simulink model "SledUnit_Levitation_Control"  (R2025a)
settings: Solver=ode23t  StartTime=0.0  StopTime=T_sim  FixedStep=0.0001  RelTol=1e-3
PreLoadFcn:
  | setup_sim_params
model workspace: external: MATLAB File .\Setup_Machine_Model\setup_structure_params.m (data not in the file)
values from neighbouring files (symbols this model uses):
  N = numel(time)    [evaluation_sled_levitation.m]
  noise_switch = 1    [setup_sim_params.m]
undefined symbols (not defined in the file or in its folder): CartJointInit, obs_init_state, obs_params, SledUnitMass, ssc_params, SUInitPosAtt2SlGCS, X, Y, Z
libraries: sm_lib x51, nesl_utility x4
(part 1 of 3)
settings Model: NumberOfSteps=3  Creator=Polarstern  LastModifiedBy=CelestialAurora
settings DataIOCC: SaveOutput=off
settings ExplorerConfigSet: SimMechanicsOpenEditorOnUpdate=off
settings ExplorerConfigSet: InternalSimMechanicsExplorerSettings=|
  | <ExplorerConfiguration>
  | 
  |   <canonicalview>planar_xy</canonicalview>
  | 
  |   <TilePanel>
  |     <TileInfo>
  |       <Tiles Columns="1" Count="1" Height="608" Rows="1" Width="1079">
  |         <Row Weight="1"/>
  |         <Column Weight="1"/>
  |         <Tile Height="1" Width="1" X="0" Y="0"/>
  |       </Tiles>
  |     </TileInfo>
  |     <SceneInfo>
  |       <SceneViewer>
  |         <IsThisViewStd>
  |           <IsStandardView>off</IsStandardView>
  |           <StandardViewName>Front</StandardViewName>
  |         </IsThisViewStd>
  |         <BGColor>
  |           <R>1</R>
  |           <G>1</G>
  |           <B>1</B>
  |           <A>1</A>
  |         </BGColor>
  |         <Camera>
  |           <DoPerspective>off</DoPerspective>
  |           <Position>
  |             <X>0.093469102418852493</X>
  |             <Y>0.022043424721416197</Y>
  |             <Z>11.197877009761701</Z>
  |           </Position>
  |           <Center>
  |             <X>0.093469102418852493</X>
  |             <Y>0.022043424721416197</Y>
  |             <Z>1.2744981024265289</Z>
  |           </Center>
  |           <Up>
  |             <X>0</X>
  |             <Y>1</Y>
  |             <Z>0</Z>
  |           </Up>
  |           <XLim>0.23710801149158423</XLim>
  |           <YLim>0.23710801149158423</YLim>
  |           <ViewLimDist>0.01</ViewLimDist>
  |         </Camera>
  |       </SceneViewer>
  |     </SceneInfo>
  |   </TilePanel>
  | 
  |   <MechEditorPanel>
  |     <GfxPanelCameraMap/>
  |     <Cameras/>
  |     <VideoCreator>
  |       <IncludeTiles>All</IncludeTiles>
  |       <IncludeTime>on</IncludeTime>
  |       <IncludeWorldFrame>off</IncludeWorldFrame>
  |       <PlaybackSpeedRatio>1</PlaybackSpeedRatio>
  |       <FrameRate>30</FrameRate>
  |       <FrameSize>auto</FrameSize>
  |       <VideoFormat>UncompressedAVI</VideoFormat>
  |     </VideoCreator>
  |   </MechEditorPanel>
  | 
  |   <PlaybackSettings>
  |     <PlaybackSpeedFactor>0.25</PlaybackSpeedFactor>
  |   </PlaybackSettings>
  | 
  | </ExplorerConfiguration>

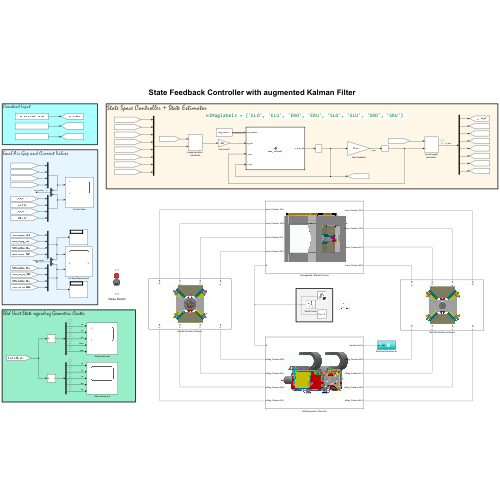
[thumbnail: Simulink's stored preview of the top-level diagram]
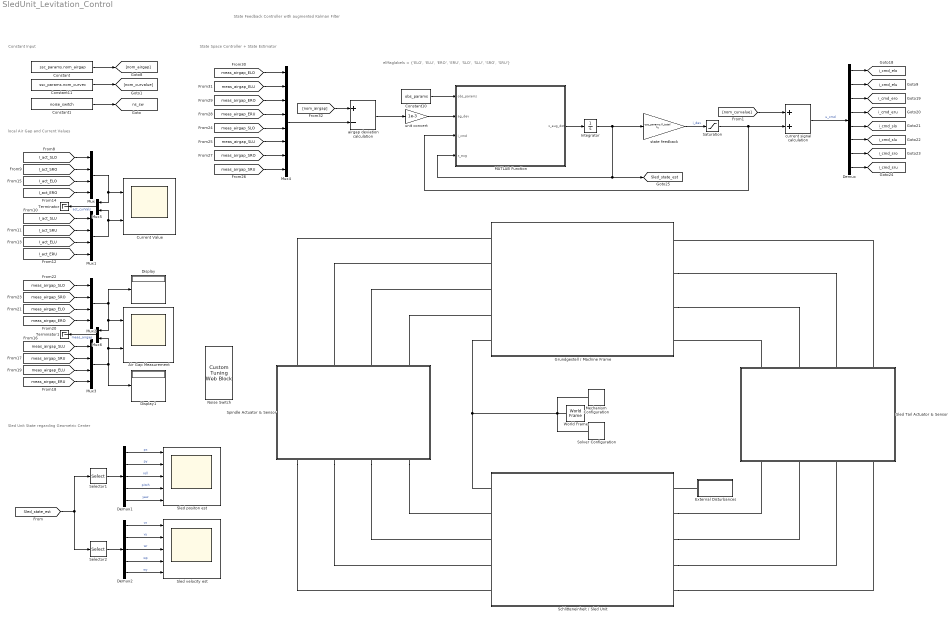
== system SledUnit_Levitation_Control ==
  note: Sled Unit State regarding Geometric Center
  note: State Space Controller + State Estimator
  note: elMaglabels = {'ELO', 'ELU', 'ERO', 'ERU', 'SLO', 'SLU', 'SRO', 'SRU'}
  note: Constant Input
  note: local Air Gap and Current Values
  note: State Feedback Controller with augmented Kalman Filter
  Air Gap Measurement : Scope  NumInputPorts=2
      settings: ActiveDisplayYMinimum=0.43274901204317934  ActiveDisplayYMaximum=0.52575342044124662  YLabel=mm
  Constant : Constant  Value=ssc_params.nom_airgap
  Constant1 : Constant  Value=noise_switch
  Constant10 : Constant  Value=obs_params  OutDataTypeStr=Bus: obs_Bus
  Constant11 : Constant  Value=ssc_params.nom_curvec
  Current Value : Scope  NumInputPorts=2
      settings: ActiveDisplayYMinimum=8.21336168307043  ActiveDisplayYMaximum=15.633373377132628
  Demux : Demux  Outputs=8
  Demux1 : Demux  Outputs=5
  Demux2 : Demux  Outputs=5
  Display : Display
  Display1 : Display
  External Disturbances : Subsystem
  Grundgestell / Machine Frame : Subsystem
      mask Display: image('.\BlockMaskIcons\machine_stand.png', [0,0,0,0,70,70]);
  Integrator : Integrator  InitialCondition=obs_init_state
  MATLAB Function : MATLAB Function  TreatAsAtomicUnit=on
  Mechanism Configuration : sm_lib/Utilities/Mechanism Configuration  UniformGravity=Constant  GravityVector=grav  GravityVectorUnits=m/s^2  LinearizationDelta=0.001  JointModeTransitionNonlinearIterations=2
  Mux{,1..3} (4 alike) : Mux
  Mux4 : Mux  Inputs=8
  Mux5 : Mux  Inputs=2
  Mux6 : Mux  Inputs=2
  Noise Switch : CustomTuningWebBlock  LabelPosition=Hide  ShowInitialText=on  Configuration="{\"components\":[{\"name\":\"CustomSwitchStateComponent\",\"settings\":{\"position\":[0,0,1,1],\"showAllLabels\":1,\"states\":[{\"HitRegion\":{\"position\":[0.5,0,1,0.5]},\"Image\":{\"position\":[0,0.24928571428571428,0.5014285714285714,1],\"size\":[0.5014285714285714,1],\"src\":\"data:image\\/svg+xml;base64,PHN2ZyB4bWxucz0iaHR0cDovL3d3dy53My5vcmcvMjAwMC9zdmciIHhtbG5zOnhsaW5rPSJodHRwOi8vd3d3LnczLm9yZy8xOTk5L3hsaW5rIiB2aWV3Qm94PSIwIDAgMzguMDQgMTUwIj48ZGVmcz48c3R5bGU+LmNscy0xe2ZpbGw6dXJsKCNyYWRpYWwtZ3JhZGllbnQpO30uY2xzLTJ7ZmlsbDp1cmwoI3JhZGlhbC1ncmFkaWVudC0yKTt9LmNscy0ze2ZpbGw6dXJsKCNXaGl0ZV9CbGFjayk7fS5jbHMtNHtmaWxsOnVybCgjcmFkaWFsLWdyYWRpZW50LTMpO30uY2xzLTV7ZmlsbDojNWI1YjViO30uY2xzLTZ7ZmlsbDp1cmwoI3Jh ...(+3556 chars)\",\"srcOrientation\":\"Right\"},\"Label\":{\"color\":[0.5019607843137255,0.5019607843137255,0.5019607843137255],\"icon\":{\"size\":[0,0],\"src\":[],\"srcOrientation\":\"Right\"},\"iconOffset\":0,\"iconPlacement\":\"left\",\"opacity\":1,\"position\":[0.92,0.5],\"show\":true,\"text\":{\"content\":\"Off\",\"font\":\"Helvetica\"}},\"Value\":0},{\"HitRegion\":{\"position\":[0,0,1,0.5]},\"Image\":{\"position\":[0,0.24928571428571428,0.5014285714285714,1],\"size\":[0.5014285714285714,1],\"src\":\"data:image\\/svg+xml;base64,PHN2ZyB4bWxucz0iaHR0cDovL3d3dy53My5vcmcvMjAwMC9zdmciIHhtbG5zOnhsaW5rPSJodHRwOi8vd3d3LnczLm9yZy8xOTk5L3hsaW5rIiB2aWV3Qm94PSIwIDAgMzguMDQgMTUwIj48ZGVmcz48c3R5bGU+LmNscy0xe2ZpbGw6dXJsKCNyYWRpYWwtZ3JhZGllbnQpO30uY2xzLTJ7ZmlsbDp1cmwoI3JhZGlhbC1ncmFkaWVudC0yKTt9LmNscy0ze2ZpbGw6dXJsKCNXaGl0ZV9CbGFjayk7fS5jbHMtNHtmaWxsOnVybCgjcmFkaWFsLWdyYWRpZW50LTMpO30uY2xzLTV7ZmlsbDojNWI1YjViO30uY2xzLTZ7ZmlsbDp1cmwoI3Jh ...(+3628 chars)\",\"srcOrientation\":\"Right\"},\"Label\":{\"color\":[0.5019607843137255,0.5019607843137255,0.5019607843137255],\"icon\":{\"size\":[0,0],\"src\":[],\"srcOrientation\":\"Right\"},\"iconOffset\":0,\"iconPlacement\":\"left\",\"opacity\":1,\"position\":[0.08,0.5],\"show\":true,\"text\":{\"content\":\"On\",\"font\":\"Helvetica\"}},\"Value\":1}]}},{\"name\":\"BackgroundImageComponent\",\"settings\":{\"image\":{\"size\":[70,135],\"src\":\"default\",\"srcOrientation\":\"Right\"},\"position\":[0,0,1,1],\"scaleMode\":\"0\"}},{\"name\":\"ForegroundImageComponent\",\"settings\":{\"image\":{\"size\":[0,0],\"src\":\"default\",\"srcOrientation\":[]},\"isForeground\":1,\"position\":[0,0,1,1],\"scaleMode\":\"0\"}}],\"derived\":{\"blockParameters\":{\"StatesJSON\":[{\"Label\":\"Off\",\"Value\":0},{\"Label\":\"On\",\"Value\":1}],\"fixedAspectRatio\":\"on\"}},\"settings\":{\"BindingType\":\"param\",\"backgroundColor\":[0,0,0],\"backgroundOffset\":0.14,\"fixedAspectRatio\":\"on\",\"foregroundColor\":[0,0,0],\"showBackgroundColor\":false,\"variant\":\"toggle\",\"version\":\"R2024b\"},\"type\":\"Switch\"}"
  Saturation : Saturate  UpperLimit=I_max - ssc_params.nom_curvec  LowerLimit=I_min - ssc_params.nom_curvec
  Schlitteneinheit / Sled Unit : Subsystem
      mask Display: image('.\BlockMaskIcons\sled_unit.png', [0,0,0,0,70,70]);
  Selector1 : Selector  InputPortWidth=ssc_params.dim_aug*1  IndexOptions=Index vector (dialog)  Indices=1:ssc_params.dim_s  OutputSizes=1
  Selector2 : Selector  InputPortWidth=ssc_params.dim_aug*1  IndexOptions=Index vector (dialog)  Indices=ssc_params.dim_s+1: ssc_params.dim_x  OutputSizes=1
  Sled Tail Actuator & Sensor : Subsystem
      mask Display: image('.\BlockMaskIcons\outer_end_face.png', [0,0,0,0,75,75]);
  Sled positon est : Scope  NumInputPorts=5
      settings: ActiveDisplayYMinimum=-2.8701521863632798E-6  ActiveDisplayYMaximum=3.1890705699246094E-7  DataLoggingVariableName=ScopeData2
  Sled velocity est : Scope  NumInputPorts=5
      settings: ActiveDisplayString=5  ActiveDisplayYMinimum=-1.0420826421465863E-6  ActiveDisplayYMaximum=1.2920620717593074E-7  DataLoggingVariableName=ScopeData3
  Solver Configuration : nesl_utility/Solver Configuration  PhysicalDomain=network_engine_domain  SubClassName=solver  LeftPortType=input  RightPortType=generic  Tones=[]  Harmonics=[]  SimulateNoise=off  Profile=off  UseLocalSampling=off  EnableSwitchedLinearOptims=on  FrequencyDomain=off  UseCCode=off  RelTol=0.001  AbsTol=0.001  MinStep=1e-09  ToWorkspace=off  RevertToSquareIcSolve=off  NumHomotopyIterations=100  PhasorMode=off  PhasorModeNumHarmonics=1  ConsistencySolver=NEWTON_XTOL_AFTER_FTOL  IndexReductionMethod=DerivativeReplacement  DoDC=off  ResidualTolerance=1e-09  ConsistencyTolSource=GLOBAL  ConsistencyAbsTol=0.001  ConsistencyRelTol=0.001  ConsistencyTolFactor=0.001  UseLocalSolver=off  LocalSolverChoice=NE_BACKWARD_EULER_ADVANCER  ResolveIndetEquations=on  FunctionEvalNumThread=1  LocalSolverSampleTime=0.001  DoFixedCost=off  MaxNonlinIter=3  MaxModeIter=2  ComputeImpulses=off  ImpulseIterations=2  LinearAlgebra=auto  LinearAlgebraNumThread=0  EquationFormulation=NE_TIME_EF  DelaysMemoryBudget=1024  AutomaticFiltering=on  FilteringTimeConstant=0.001  PartitionStorageMethod=AS_NEEDED  PartitionMemoryBudget=1024  PartitionMethod=ROBUST  MultibodyUseLocalSolver=off  MultibodyLocalSolverChoice=ODE1  MultibodyLocalSolverSampleTime=0.001
  Spindle Actuator & Sensor : Subsystem
      mask Display: image('.\BlockMaskIcons\spindle_end_face.png', [0,0,0,0,75,75]);
  Terminator : Terminator
  Terminator1 : Terminator
  World Frame : sm_lib/Frames and Transforms/World Frame
  airgap deviation calculation : Sum  Inputs=+-  OutDataTypeStr=double
  "current signal calculation " : Sum
  state feedback : Gain  Gain=-ssc_params.K_total  Multiplication=Matrix(K*u) (u vector)
  unit convert : Gain  Gain=1e-3
  tag scope: Sled_state_est=global, i_cmd_elo=global, i_cmd_elu=global, i_cmd_ero=global, i_cmd_eru=global, i_cmd_slo=global, i_cmd_slu=global, i_cmd_sro=global, i_cmd_sru=global, ns_sw=global
  wires:
  [I_act_ELO] -> Mux/3
  [I_act_SRO] -> Mux/2
  [I_act_SLO] -> Mux/1
  [I_act_ERO] -> Mux/4
  [I_act_SLU] -> Mux1/1
  [I_act_SRU] -> Mux1/2
  [I_act_ELU] -> Mux1/3
  [I_act_ERU] -> Mux1/4
  Mux/1 -> Mux5/1, Current Value/1
  Mux1/1 -> Mux5/2, Current Value/2
  Mux2/1 -> Mux6/1, Air Gap Measurement/1, Display/1
  [meas_airgap_ERU] -> Mux3/4
  [meas_airgap_SLU] -> Mux3/1
  Mux3/1 -> Display1/1, Mux6/2, Air Gap Measurement/2
  [meas_airgap_SLO] -> Mux2/1
  [meas_airgap_SRO] -> Mux2/2
  [meas_airgap_ERO] -> Mux2/4
  [meas_airgap_ELO] -> Mux2/3
  [meas_airgap_ELU] -> Mux3/3
  [meas_airgap_SRU] -> Mux3/2
  Constant/1 -> [nom_airgap]
  Demux/1 -> [i_cmd_elo]
  [meas_airgap_ELO] -> Mux4/1
  [meas_airgap_ELU] -> Mux4/2
  [meas_airgap_ERO] -> Mux4/3
  [meas_airgap_ERU] -> Mux4/4
  [meas_airgap_SLO] -> Mux4/5
  [meas_airgap_SLU] -> Mux4/6
  [meas_airgap_SRO] -> Mux4/7
  [meas_airgap_SRU] -> Mux4/8
  Demux/2 -> [i_cmd_elu]
  Demux/3 -> [i_cmd_ero]
  Demux/4 -> [i_cmd_eru]
  Demux/5 -> [i_cmd_slo]
  Demux/6 -> [i_cmd_slu]
  Demux/7 -> [i_cmd_sro]
  Demux/8 -> [i_cmd_sru]
  Mux4/1 -> airgap deviation calculation/2
  [nom_airgap] -> airgap deviation calculation/1
  airgap deviation calculation/1 -> unit convert/1
  [Sled_state_est] -> Selector2/1, Selector1/1
  Selector1/1 -> Demux1/1
  Demux1/3 -> Sled positon est/3  "roll"
  Demux1/1 -> Sled positon est/1  "px"
  Demux1/2 -> Sled positon est/2  "py"
  Demux1/4 -> Sled positon est/4  "pitch"
  Demux1/5 -> Sled positon est/5  "yaw"
  Demux2/2 -> Sled velocity est/2  "vy"
  Demux2/1 -> Sled velocity est/1  "vx"
  Demux2/5 -> Sled velocity est/5  "wy"
  Demux2/4 -> Sled velocity est/4  "wp"
  Demux2/3 -> Sled velocity est/3  "wr"
  Selector2/1 -> Demux2/1
  [nom_curvalue] -> "current signal calculation "/1
  Constant11/1 -> [nom_curvalue]
  Constant1/1 -> [ns_sw]
  "current signal calculation "/1 -> Demux/1  "u_cmd"
  Mux5/1 -> Terminator/1  "act_curVals"
  Mux6/1 -> Terminator1/1  "meas_airgap"
  Integrator/1 -> MATLAB Function/4(x_aug), [Sled_state_est], state feedback/1
  state feedback/1 -> Saturation/1  "i_dev"
  Saturation/1 -> "current signal calculation "/2, MATLAB Function/3(i_cmd)
  Constant10/1 -> MATLAB Function/1(obs_params)
  unit convert/1 -> MATLAB Function/2(ag_dev)
  MATLAB Function/1(x_aug_dot) -> Integrator/1
  connections:
  Mechanism Configuration/RConn1 -- Grundgestell / Machine Frame/LConn5 -- Schlitteneinheit / Sled Unit/LConn1 -- Solver Configuration/RConn1 -- World Frame/RConn1
  External Disturbances/RConn1 -- Schlitteneinheit / Sled Unit/RConn1
  Grundgestell / Machine Frame/LConn4 -- Spindle Actuator & Sensor/RConn4
  Grundgestell / Machine Frame/LConn3 -- Spindle Actuator & Sensor/RConn3
  Grundgestell / Machine Frame/LConn2 -- Spindle Actuator & Sensor/RConn2
  Grundgestell / Machine Frame/LConn1 -- Spindle Actuator & Sensor/RConn1
  Spindle Actuator & Sensor/LConn4 -- Schlitteneinheit / Sled Unit/LConn2
  Spindle Actuator & Sensor/LConn3 -- Schlitteneinheit / Sled Unit/LConn3
  Spindle Actuator & Sensor/LConn2 -- Schlitteneinheit / Sled Unit/LConn4
  Spindle Actuator & Sensor/LConn1 -- Schlitteneinheit / Sled Unit/LConn5
  Sled Tail Actuator & Sensor/RConn1 -- Grundgestell / Machine Frame/RConn4
  Grundgestell / Machine Frame/RConn3 -- Sled Tail Actuator & Sensor/RConn2
  Grundgestell / Machine Frame/RConn2 -- Sled Tail Actuator & Sensor/RConn3
  Sled Tail Actuator & Sensor/RConn4 -- Grundgestell / Machine Frame/RConn1
  Schlitteneinheit / Sled Unit/RConn2 -- Sled Tail Actuator & Sensor/LConn1
  Schlitteneinheit / Sled Unit/RConn3 -- Sled Tail Actuator & Sensor/LConn2
  Schlitteneinheit / Sled Unit/RConn4 -- Sled Tail Actuator & Sensor/LConn3
  Schlitteneinheit / Sled Unit/RConn5 -- Sled Tail Actuator & Sensor/LConn4

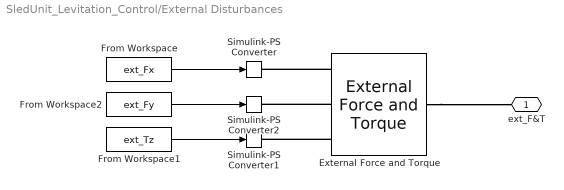
== system SledUnit_Levitation_Control/External Disturbances ==
  External Force and Torque : sm_lib/Forces and Torques/External Force and Torque  EnableForceX=on  EnableForceY=on  EnableForceZ=off  EnableForce=off  ForceResolutionFrame=AttachedFrame  EnableTorqueX=off  EnableTorqueY=off  EnableTorqueZ=on  EnableTorque=off  TorqueResolutionFrame=AttachedFrame
  From Workspace : FromWorkspace  VariableName=ext_Fx  OutDataTypeStr=double
  From Workspace1 : FromWorkspace  VariableName=ext_Tz  OutDataTypeStr=double
  From Workspace2 : FromWorkspace  VariableName=ext_Fy  OutDataTypeStr=double
  Simulink-PS Converter : nesl_utility/Simulink-PS Converter  PhysicalDomain=network_engine_domain  SubClassName=ps_input  LeftPortType=input  RightPortType=output  PseudoPeriodic=off  Frequencies=[]  NoiseDistribution=none  NoiseParameters=[]  Unit=1  AffineConversion=off  FilteringAndDerivatives=provide  SimscapeFilterOrder=1  InputFilterTimeConstant=0.001  UdotUserProvided=0
  Simulink-PS Converter1 : nesl_utility/Simulink-PS Converter  PhysicalDomain=network_engine_domain  SubClassName=ps_input  LeftPortType=input  RightPortType=output  PseudoPeriodic=off  Frequencies=[]  NoiseDistribution=none  NoiseParameters=[]  Unit=N*m  AffineConversion=on  FilteringAndDerivatives=provide  SimscapeFilterOrder=1  InputFilterTimeConstant=0.001  UdotUserProvided=0
  Simulink-PS Converter2 : nesl_utility/Simulink-PS Converter  PhysicalDomain=network_engine_domain  SubClassName=ps_input  LeftPortType=input  RightPortType=output  PseudoPeriodic=off  Frequencies=[]  NoiseDistribution=none  NoiseParameters=[]  Unit=1  AffineConversion=off  FilteringAndDerivatives=provide  SimscapeFilterOrder=1  InputFilterTimeConstant=0.001  UdotUserProvided=0
  ext_F&T : PMIOPort  Side=Right
  wires:
  From Workspace/1 -> Simulink-PS Converter/1
  From Workspace1/1 -> Simulink-PS Converter1/1
  From Workspace2/1 -> Simulink-PS Converter2/1
  connections:
  External Force and Torque/RConn1 -- ext_F&T/RConn1
  External Force and Torque/LConn1 -- Simulink-PS Converter/RConn1
  External Force and Torque/LConn3 -- Simulink-PS Converter1/RConn1
  External Force and Torque/LConn2 -- Simulink-PS Converter2/RConn1

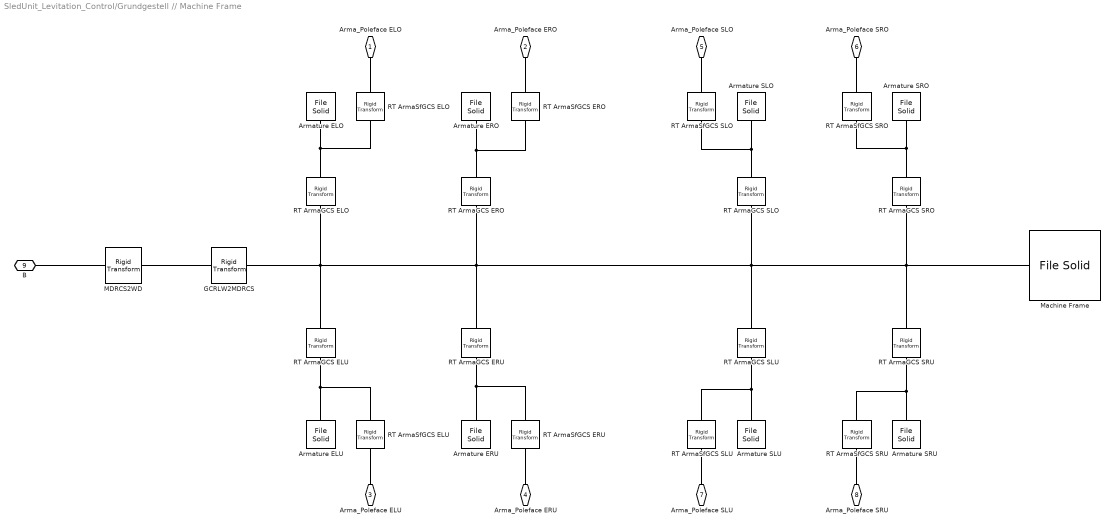
== system SledUnit_Levitation_Control/Grundgestell // Machine Frame ==
  Armature ELO : sm_lib/Body Elements/File Solid  ExtGeomFileName=.\Simplified_CAD_Model\Magnetschiene_rechts.stp  UnitType=Custom  ExtGeomFileUnits=mm  StepReaderType=HEX  ExportConvexHullGeometry=off  InertiaType=Custom  BasedOnType=Density  Density=1000  DensityUnits=kg/m^3  Mass=32.666  MassUnits=kg  CenterOfMass=[0 0 0]  CenterOfMassUnits=m  MomentsOfInertia=[1 1 1]  MomentsOfInertiaUnits=kg*m^2  ProductsOfInertia=[0 0 0]  ProductsOfInertiaUnits=kg*m^2  GraphicType=FromGeometry  MarkerShape=Sphere  MarkerSize=10  GraphicVisPropType=SimpleVisualProperties  GraphicDiffuseColor=[0.2706 0.4039 0.7137]  GraphicOpacity=1  GraphicSpecularColor=[0.5 0.5 0.5 1.0]  GraphicAmbientColor=[0.15 0.15 0.15 1.0]  GraphicEmissiveColor=[0.0 0.0 0.0 1.0]  GraphicShininess=75  DoExposeReferenceFrame=on  SerializedFrames=<Frames/>
  Armature ELU : sm_lib/Body Elements/File Solid  ExtGeomFileName=.\Simplified_CAD_Model\Magnetschiene_links.stp  UnitType=Custom  ExtGeomFileUnits=mm  StepReaderType=HEX  ExportConvexHullGeometry=off  InertiaType=Custom  BasedOnType=Density  Density=1.002  DensityUnits=g/cm^3  Mass=32.666  MassUnits=kg  CenterOfMass=[0 0 0]  CenterOfMassUnits=m  MomentsOfInertia=[1 1 1]  MomentsOfInertiaUnits=kg*m^2  ProductsOfInertia=[0 0 0]  ProductsOfInertiaUnits=kg*m^2  GraphicType=FromGeometry  MarkerShape=Sphere  MarkerSize=10  GraphicVisPropType=SimpleVisualProperties  GraphicDiffuseColor=[0.2706 0.4039 0.7137]  GraphicOpacity=1  GraphicSpecularColor=[0.5 0.5 0.5 1.0]  GraphicAmbientColor=[0.15 0.15 0.15 1.0]  GraphicEmissiveColor=[0.0 0.0 0.0 1.0]  GraphicShininess=75  DoExposeReferenceFrame=on  SerializedFrames=<Frames/>
  Armature ERO : sm_lib/Body Elements/File Solid  ExtGeomFileName=.\Simplified_CAD_Model\Magnetschiene_links.stp  UnitType=Custom  ExtGeomFileUnits=mm  StepReaderType=HEX  ExportConvexHullGeometry=off  InertiaType=Custom  BasedOnType=DensityFromFile  Density=1000  DensityUnits=kg/m^3  Mass=32.666  MassUnits=kg  CenterOfMass=[0 0 0]  CenterOfMassUnits=m  MomentsOfInertia=[1 1 1]  MomentsOfInertiaUnits=kg*m^2  ProductsOfInertia=[0 0 0]  ProductsOfInertiaUnits=kg*m^2  GraphicType=FromGeometry  MarkerShape=Sphere  MarkerSize=10  GraphicVisPropType=SimpleVisualProperties  GraphicDiffuseColor=[0.2706 0.4039 0.7137]  GraphicOpacity=1  GraphicSpecularColor=[0.5 0.5 0.5 1.0]  GraphicAmbientColor=[0.15 0.15 0.15 1.0]  GraphicEmissiveColor=[0.0 0.0 0.0 1.0]  GraphicShininess=75  DoExposeReferenceFrame=on  SerializedFrames=<Frames/>
  Armature ERU : sm_lib/Body Elements/File Solid  ExtGeomFileName=.\Simplified_CAD_Model\Magnetschiene_rechts.stp  UnitType=Custom  ExtGeomFileUnits=mm  StepReaderType=HEX  ExportConvexHullGeometry=off  InertiaType=Custom  BasedOnType=DensityFromFile  Density=1000  DensityUnits=kg/m^3  Mass=32.666  MassUnits=kg  CenterOfMass=[0 0 0]  CenterOfMassUnits=m  MomentsOfInertia=[1 1 1]  MomentsOfInertiaUnits=kg*m^2  ProductsOfInertia=[0 0 0]  ProductsOfInertiaUnits=kg*m^2  GraphicType=FromGeometry  MarkerShape=Sphere  MarkerSize=10  GraphicVisPropType=SimpleVisualProperties  GraphicDiffuseColor=[0.2706 0.4039 0.7137]  GraphicOpacity=1  GraphicSpecularColor=[0.5 0.5 0.5 1.0]  GraphicAmbientColor=[0.15 0.15 0.15 1.0]  GraphicEmissiveColor=[0.0 0.0 0.0 1.0]  GraphicShininess=75  DoExposeReferenceFrame=on  SerializedFrames=<Frames/>
  Armature SLO : sm_lib/Body Elements/File Solid  ExtGeomFileName=.\Simplified_CAD_Model\Magnetschiene_links.stp  UnitType=Custom  ExtGeomFileUnits=mm  StepReaderType=HEX  ExportConvexHullGeometry=off  InertiaType=Custom  BasedOnType=DensityFromFile  Density=1000  DensityUnits=kg/m^3  Mass=32.666  MassUnits=kg  CenterOfMass=[0 0 0]  CenterOfMassUnits=m  MomentsOfInertia=[1 1 1]  MomentsOfInertiaUnits=kg*m^2  ProductsOfInertia=[0 0 0]  ProductsOfInertiaUnits=kg*m^2  GraphicType=FromGeometry  MarkerShape=Sphere  MarkerSize=10  GraphicVisPropType=SimpleVisualProperties  GraphicDiffuseColor=[0.2706 0.4039 0.7137]  GraphicOpacity=1  GraphicSpecularColor=[0.5 0.5 0.5 1.0]  GraphicAmbientColor=[0.15 0.15 0.15 1.0]  GraphicEmissiveColor=[0.0 0.0 0.0 1.0]  GraphicShininess=75  DoExposeReferenceFrame=on  SerializedFrames=<Frames/>
  Armature SLU : sm_lib/Body Elements/File Solid  ExtGeomFileName=.\Simplified_CAD_Model\Magnetschiene_rechts.stp  UnitType=Custom  ExtGeomFileUnits=mm  StepReaderType=HEX  ExportConvexHullGeometry=off  InertiaType=Custom  BasedOnType=Mass  Density=1.002  DensityUnits=g/cm^3  Mass=32.666  MassUnits=kg  CenterOfMass=[0 0 0]  CenterOfMassUnits=m  MomentsOfInertia=[1 1 1]  MomentsOfInertiaUnits=kg*m^2  ProductsOfInertia=[0 0 0]  ProductsOfInertiaUnits=kg*m^2  GraphicType=FromGeometry  MarkerShape=Sphere  MarkerSize=10  GraphicVisPropType=SimpleVisualProperties  GraphicDiffuseColor=[0.2706 0.4039 0.7137]  GraphicOpacity=1  GraphicSpecularColor=[0.5 0.5 0.5 1.0]  GraphicAmbientColor=[0.15 0.15 0.15 1.0]  GraphicEmissiveColor=[0.0 0.0 0.0 1.0]  GraphicShininess=75  DoExposeReferenceFrame=on  SerializedFrames=<Frames/>
  Armature SRO : sm_lib/Body Elements/File Solid  ExtGeomFileName=.\Simplified_CAD_Model\Magnetschiene_rechts.stp  UnitType=Custom  ExtGeomFileUnits=mm  StepReaderType=HEX  ExportConvexHullGeometry=off  InertiaType=Custom  BasedOnType=DensityFromFile  Density=1000  DensityUnits=kg/m^3  Mass=32.666  MassUnits=kg  CenterOfMass=[0 0 0]  CenterOfMassUnits=m  MomentsOfInertia=[1 1 1]  MomentsOfInertiaUnits=kg*m^2  ProductsOfInertia=[0 0 0]  ProductsOfInertiaUnits=kg*m^2  GraphicType=FromGeometry  MarkerShape=Sphere  MarkerSize=10  GraphicVisPropType=SimpleVisualProperties  GraphicDiffuseColor=[0.2706 0.4039 0.7137]  GraphicOpacity=1  GraphicSpecularColor=[0.5 0.5 0.5 1.0]  GraphicAmbientColor=[0.15 0.15 0.15 1.0]  GraphicEmissiveColor=[0.0 0.0 0.0 1.0]  GraphicShininess=75  DoExposeReferenceFrame=on  SerializedFrames=<Frames/>
  Armature SRU : sm_lib/Body Elements/File Solid  ExtGeomFileName=.\Simplified_CAD_Model\Magnetschiene_links.stp  UnitType=Custom  ExtGeomFileUnits=mm  StepReaderType=HEX  ExportConvexHullGeometry=off  InertiaType=Custom  BasedOnType=DensityFromFile  Density=1000  DensityUnits=kg/m^3  Mass=32.666  MassUnits=kg  CenterOfMass=[0 0 0]  CenterOfMassUnits=m  MomentsOfInertia=[1 1 1]  MomentsOfInertiaUnits=kg*m^2  ProductsOfInertia=[0 0 0]  ProductsOfInertiaUnits=kg*m^2  GraphicType=FromGeometry  MarkerShape=Sphere  MarkerSize=10  GraphicVisPropType=SimpleVisualProperties  GraphicDiffuseColor=[0.2706 0.4039 0.7137]  GraphicOpacity=1  GraphicSpecularColor=[0.5 0.5 0.5 1.0]  GraphicAmbientColor=[0.15 0.15 0.15 1.0]  GraphicEmissiveColor=[0.0 0.0 0.0 1.0]  GraphicShininess=75  DoExposeReferenceFrame=on  SerializedFrames=<Frames/>
  GCRLW2MDRCS : sm_lib/Frames and Transforms/Rigid Transform  RotationMethod=RotationSequence  FollAlignAxisA=+X  BaseAlignAxisA=+Y  FollAlignAxisB=+Y  BaseAlignAxisB=+Z  RotationStandardAxis=+Z  RotationAngle=0  RotationAngleUnits=deg  RotationArbitraryAxis=[0 0 1]  RotationSequenceAxes=FollowerAxes  RotationSequence=ZYX  RotationSequenceAngles=GCRLW2MDRCS.RA  RotationSequenceAnglesUnits=rad  RotationMatrix=[1 0 0;0 1 0;0 0 1]  Quaternion=[1 0 0 0]  TranslationMethod=Cartesian  TranslationCartesianOffset=GCRLW2MDRCS.TV  TranslationCartesianOffsetUnits=mm  TranslationStandardAxis=+Z  TranslationStandardOffset=0  TranslationStandardOffsetUnits=m  TranslationROffset=0  TranslationROffsetUnits=m  TranslationThetaOffset=0  TranslationThetaOffsetUnits=deg  TranslationZOffset=0  TranslationZOffsetUnits=m
  MDRCS2WD : sm_lib/Frames and Transforms/Rigid Transform  RotationMethod=None  FollAlignAxisA=+X  BaseAlignAxisA=+Y  FollAlignAxisB=+Y  BaseAlignAxisB=+Z  RotationStandardAxis=+Z  RotationAngle=0  RotationAngleUnits=deg  RotationArbitraryAxis=[0 0 1]  RotationSequenceAxes=FollowerAxes  RotationSequence=XYX  RotationSequenceAngles=[0 0 0]  RotationSequenceAnglesUnits=deg  RotationMatrix=[1 0 0;0 1 0;0 0 1]  Quaternion=[1 0 0 0]  TranslationMethod=None  TranslationCartesianOffset=[0 0 0]  TranslationCartesianOffsetUnits=m  TranslationStandardAxis=+Z  TranslationStandardOffset=0  TranslationStandardOffsetUnits=m  TranslationROffset=0  TranslationROffsetUnits=m  TranslationThetaOffset=0  TranslationThetaOffsetUnits=deg  TranslationZOffset=0  TranslationZOffsetUnits=m
  Machine Frame : sm_lib/Body Elements/File Solid  ExtGeomFileName=.\Simplified_CAD_Model\Grundgestell.stp  UnitType=Custom  ExtGeomFileUnits=mm  StepReaderType=HEX  ExportConvexHullGeometry=off  InertiaType=Custom  BasedOnType=DensityFromFile  Density=100000  DensityUnits=kg/m^3  Mass=100000  MassUnits=kg  CenterOfMass=[0 0 0]  CenterOfMassUnits=mm  MomentsOfInertia=[1 1 1]  MomentsOfInertiaUnits=kg*m^2  ProductsOfInertia=[0 0 0]  ProductsOfInertiaUnits=kg*m^2  GraphicType=FromGeometry  MarkerShape=Sphere  MarkerSize=10  GraphicVisPropType=SimpleVisualProperties  GraphicDiffuseColor=[0.5098 0.5098 0.5098]  GraphicOpacity=1  GraphicSpecularColor=[0.5 0.5 0.5 1.0]  GraphicAmbientColor=[0.15 0.15 0.15 1.0]  GraphicEmissiveColor=[0.0 0.0 0.0 1.0]  GraphicShininess=75  DoExposeReferenceFrame=on  SerializedFrames=<Frames/>
  RT ArmaGCS ELO : sm_lib/Frames and Transforms/Rigid Transform  RotationMethod=RotationSequence  FollAlignAxisA=+X  BaseAlignAxisA=+Y  FollAlignAxisB=+Y  BaseAlignAxisB=+Z  RotationStandardAxis=+Z  RotationAngle=0  RotationAngleUnits=deg  RotationArbitraryAxis=[0 0 1]  RotationSequenceAxes=FollowerAxes  RotationSequence=ZYX  RotationSequenceAngles=ArmaGCF2GCRLW.ELO.RA  RotationSequenceAnglesUnits=rad  RotationMatrix=[1 0 0;0 1 0;0 0 1]  Quaternion=[1 0 0 0]  TranslationMethod=Cartesian  TranslationCartesianOffset=ArmaGCF2GCRLW.ELO.TV  TranslationCartesianOffsetUnits=mm  TranslationStandardAxis=+Z  TranslationStandardOffset=0  TranslationStandardOffsetUnits=m  TranslationROffset=0  TranslationROffsetUnits=m  TranslationThetaOffset=0  TranslationThetaOffsetUnits=deg  TranslationZOffset=0  TranslationZOffsetUnits=m
  RT ArmaGCS ELU : sm_lib/Frames and Transforms/Rigid Transform  RotationMethod=RotationSequence  FollAlignAxisA=+X  BaseAlignAxisA=+Y  FollAlignAxisB=+Y  BaseAlignAxisB=+Z  RotationStandardAxis=+Z  RotationAngle=0  RotationAngleUnits=deg  RotationArbitraryAxis=[0 0 1]  RotationSequenceAxes=FollowerAxes  RotationSequence=ZYX  RotationSequenceAngles=ArmaGCF2GCRLW.ELU.RA  RotationSequenceAnglesUnits=rad  RotationMatrix=[1 0 0;0 1 0;0 0 1]  Quaternion=[1 0 0 0]  TranslationMethod=Cartesian  TranslationCartesianOffset=ArmaGCF2GCRLW.ELU.TV  TranslationCartesianOffsetUnits=mm  TranslationStandardAxis=+Z  TranslationStandardOffset=0  TranslationStandardOffsetUnits=m  TranslationROffset=0  TranslationROffsetUnits=m  TranslationThetaOffset=0  TranslationThetaOffsetUnits=deg  TranslationZOffset=0  TranslationZOffsetUnits=m
  RT ArmaGCS ERO : sm_lib/Frames and Transforms/Rigid Transform  RotationMethod=RotationSequence  FollAlignAxisA=+X  BaseAlignAxisA=+Y  FollAlignAxisB=+Y  BaseAlignAxisB=+Z  RotationStandardAxis=+Z  RotationAngle=0  RotationAngleUnits=deg  RotationArbitraryAxis=[0 0 1]  RotationSequenceAxes=FollowerAxes  RotationSequence=ZYX  RotationSequenceAngles=ArmaGCF2GCRLW.ERO.RA  RotationSequenceAnglesUnits=rad  RotationMatrix=[1 0 0;0 1 0;0 0 1]  Quaternion=[1 0 0 0]  TranslationMethod=Cartesian  TranslationCartesianOffset=ArmaGCF2GCRLW.ERO.TV  TranslationCartesianOffsetUnits=mm  TranslationStandardAxis=+Z  TranslationStandardOffset=0  TranslationStandardOffsetUnits=m  TranslationROffset=0  TranslationROffsetUnits=m  TranslationThetaOffset=0  TranslationThetaOffsetUnits=deg  TranslationZOffset=0  TranslationZOffsetUnits=m
  RT ArmaGCS ERU : sm_lib/Frames and Transforms/Rigid Transform  RotationMethod=RotationSequence  FollAlignAxisA=+X  BaseAlignAxisA=+Y  FollAlignAxisB=+Y  BaseAlignAxisB=+Z  RotationStandardAxis=+Z  RotationAngle=0  RotationAngleUnits=deg  RotationArbitraryAxis=[0 0 1]  RotationSequenceAxes=FollowerAxes  RotationSequence=ZYX  RotationSequenceAngles=ArmaGCF2GCRLW.ERU.RA  RotationSequenceAnglesUnits=rad  RotationMatrix=[1 0 0;0 1 0;0 0 1]  Quaternion=[1 0 0 0]  TranslationMethod=Cartesian  TranslationCartesianOffset=ArmaGCF2GCRLW.ERU.TV  TranslationCartesianOffsetUnits=mm  TranslationStandardAxis=+Z  TranslationStandardOffset=0  TranslationStandardOffsetUnits=m  TranslationROffset=0  TranslationROffsetUnits=m  TranslationThetaOffset=0  TranslationThetaOffsetUnits=deg  TranslationZOffset=0  TranslationZOffsetUnits=m
  RT ArmaGCS SLO : sm_lib/Frames and Transforms/Rigid Transform  RotationMethod=RotationSequence  FollAlignAxisA=+X  BaseAlignAxisA=+Y  FollAlignAxisB=+Y  BaseAlignAxisB=+Z  RotationStandardAxis=+Z  RotationAngle=0  RotationAngleUnits=deg  RotationArbitraryAxis=[0 0 1]  RotationSequenceAxes=FollowerAxes  RotationSequence=ZYX  RotationSequenceAngles=ArmaGCF2GCRLW.SLO.RA  RotationSequenceAnglesUnits=rad  RotationMatrix=[1 0 0;0 1 0;0 0 1]  Quaternion=[1 0 0 0]  TranslationMethod=Cartesian  TranslationCartesianOffset=ArmaGCF2GCRLW.SLO.TV  TranslationCartesianOffsetUnits=mm  TranslationStandardAxis=+Z  TranslationStandardOffset=0  TranslationStandardOffsetUnits=m  TranslationROffset=0  TranslationROffsetUnits=m  TranslationThetaOffset=0  TranslationThetaOffsetUnits=deg  TranslationZOffset=0  TranslationZOffsetUnits=m
  RT ArmaGCS SLU : sm_lib/Frames and Transforms/Rigid Transform  RotationMethod=RotationSequence  FollAlignAxisA=+X  BaseAlignAxisA=+Y  FollAlignAxisB=+Y  BaseAlignAxisB=+Z  RotationStandardAxis=+Z  RotationAngle=0  RotationAngleUnits=deg  RotationArbitraryAxis=[0 0 1]  RotationSequenceAxes=FollowerAxes  RotationSequence=ZYX  RotationSequenceAngles=ArmaGCF2GCRLW.SLU.RA  RotationSequenceAnglesUnits=rad  RotationMatrix=[1 0 0;0 1 0;0 0 1]  Quaternion=[1 0 0 0]  TranslationMethod=Cartesian  TranslationCartesianOffset=ArmaGCF2GCRLW.SLU.TV  TranslationCartesianOffsetUnits=mm  TranslationStandardAxis=+Z  TranslationStandardOffset=0  TranslationStandardOffsetUnits=m  TranslationROffset=0  TranslationROffsetUnits=m  TranslationThetaOffset=0  TranslationThetaOffsetUnits=deg  TranslationZOffset=0  TranslationZOffsetUnits=m
  RT ArmaGCS SRO : sm_lib/Frames and Transforms/Rigid Transform  RotationMethod=RotationSequence  FollAlignAxisA=+X  BaseAlignAxisA=+Y  FollAlignAxisB=+Y  BaseAlignAxisB=+Z  RotationStandardAxis=+Z  RotationAngle=0  RotationAngleUnits=deg  RotationArbitraryAxis=[0 0 1]  RotationSequenceAxes=FollowerAxes  RotationSequence=ZYX  RotationSequenceAngles=ArmaGCF2GCRLW.SRO.RA  RotationSequenceAnglesUnits=rad  RotationMatrix=[1 0 0;0 1 0;0 0 1]  Quaternion=[1 0 0 0]  TranslationMethod=Cartesian  TranslationCartesianOffset=ArmaGCF2GCRLW.SRO.TV  TranslationCartesianOffsetUnits=mm  TranslationStandardAxis=+Z  TranslationStandardOffset=0  TranslationStandardOffsetUnits=m  TranslationROffset=0  TranslationROffsetUnits=m  TranslationThetaOffset=0  TranslationThetaOffsetUnits=deg  TranslationZOffset=0  TranslationZOffsetUnits=m
  RT ArmaGCS SRU : sm_lib/Frames and Transforms/Rigid Transform  RotationMethod=RotationSequence  FollAlignAxisA=+X  BaseAlignAxisA=+Y  FollAlignAxisB=+Y  BaseAlignAxisB=+Z  RotationStandardAxis=+Z  RotationAngle=0  RotationAngleUnits=deg  RotationArbitraryAxis=[0 0 1]  RotationSequenceAxes=FollowerAxes  RotationSequence=ZYX  RotationSequenceAngles=ArmaGCF2GCRLW.SRU.RA  RotationSequenceAnglesUnits=rad  RotationMatrix=[1 0 0;0 1 0;0 0 1]  Quaternion=[1 0 0 0]  TranslationMethod=Cartesian  TranslationCartesianOffset=ArmaGCF2GCRLW.SRU.TV  TranslationCartesianOffsetUnits=mm  TranslationStandardAxis=+Z  TranslationStandardOffset=0  TranslationStandardOffsetUnits=m  TranslationROffset=0  TranslationROffsetUnits=m  TranslationThetaOffset=0  TranslationThetaOffsetUnits=deg  TranslationZOffset=0  TranslationZOffsetUnits=m
  RT ArmaSfGCS ELO : sm_lib/Frames and Transforms/Rigid Transform  RotationMethod=RotationSequence  FollAlignAxisA=+X  BaseAlignAxisA=+Y  FollAlignAxisB=+Y  BaseAlignAxisB=+Z  RotationStandardAxis=+Z  RotationAngle=0  RotationAngleUnits=deg  RotationArbitraryAxis=[0 0 1]  RotationSequenceAxes=FollowerAxes  RotationSequence=ZYX  RotationSequenceAngles=ArmaSfCS_RA.ELO  RotationSequenceAnglesUnits=rad  RotationMatrix=[1 0 0;0 1 0;0 0 1]  Quaternion=[1 0 0 0]  TranslationMethod=StandardAxis  TranslationCartesianOffset=ArmaSfCSTV2GCSRlW.ELO  TranslationCartesianOffsetUnits=mm  TranslationStandardAxis=+Y  TranslationStandardOffset=ArmaSfCS_Y_Off  TranslationStandardOffsetUnits=mm  TranslationROffset=0  TranslationROffsetUnits=m  TranslationThetaOffset=0  TranslationThetaOffsetUnits=deg  TranslationZOffset=0  TranslationZOffsetUnits=m
  RT ArmaSfGCS ELU : sm_lib/Frames and Transforms/Rigid Transform  RotationMethod=RotationSequence  FollAlignAxisA=+X  BaseAlignAxisA=+Y  FollAlignAxisB=+Y  BaseAlignAxisB=+Z  RotationStandardAxis=+Z  RotationAngle=0  RotationAngleUnits=deg  RotationArbitraryAxis=[0 0 1]  RotationSequenceAxes=FollowerAxes  RotationSequence=ZYX  RotationSequenceAngles=ArmaSfCS_RA.ELU  RotationSequenceAnglesUnits=rad  RotationMatrix=[1 0 0;0 1 0;0 0 1]  Quaternion=[1 0 0 0]  TranslationMethod=StandardAxis  TranslationCartesianOffset=[0 0 0]  TranslationCartesianOffsetUnits=m  TranslationStandardAxis=+Y  TranslationStandardOffset=ArmaSfCS_Y_Off  TranslationStandardOffsetUnits=mm  TranslationROffset=0  TranslationROffsetUnits=m  TranslationThetaOffset=0  TranslationThetaOffsetUnits=deg  TranslationZOffset=0  TranslationZOffsetUnits=m
  RT ArmaSfGCS ERO : sm_lib/Frames and Transforms/Rigid Transform  RotationMethod=RotationSequence  FollAlignAxisA=+X  BaseAlignAxisA=+Y  FollAlignAxisB=+Y  BaseAlignAxisB=+Z  RotationStandardAxis=+Z  RotationAngle=0  RotationAngleUnits=deg  RotationArbitraryAxis=[0 0 1]  RotationSequenceAxes=FollowerAxes  RotationSequence=ZYX  RotationSequenceAngles=ArmaSfCS_RA.ERO  RotationSequenceAnglesUnits=rad  RotationMatrix=[1 0 0;0 1 0;0 0 1]  Quaternion=[1 0 0 0]  TranslationMethod=StandardAxis  TranslationCartesianOffset=[0 0 0]  TranslationCartesianOffsetUnits=m  TranslationStandardAxis=+Y  TranslationStandardOffset=ArmaSfCS_Y_Off  TranslationStandardOffsetUnits=mm  TranslationROffset=0  TranslationROffsetUnits=m  TranslationThetaOffset=0  TranslationThetaOffsetUnits=deg  TranslationZOffset=0  TranslationZOffsetUnits=m
  RT ArmaSfGCS ERU : sm_lib/Frames and Transforms/Rigid Transform  RotationMethod=RotationSequence  FollAlignAxisA=+X  BaseAlignAxisA=+Y  FollAlignAxisB=+Y  BaseAlignAxisB=+Z  RotationStandardAxis=+Z  RotationAngle=0  RotationAngleUnits=deg  RotationArbitraryAxis=[0 0 1]  RotationSequenceAxes=FollowerAxes  RotationSequence=ZYX  RotationSequenceAngles=ArmaSfCS_RA.ERU  RotationSequenceAnglesUnits=rad  RotationMatrix=[1 0 0;0 1 0;0 0 1]  Quaternion=[1 0 0 0]  TranslationMethod=StandardAxis  TranslationCartesianOffset=[0 0 0]  TranslationCartesianOffsetUnits=m  TranslationStandardAxis=+Y  TranslationStandardOffset=ArmaSfCS_Y_Off  TranslationStandardOffsetUnits=mm  TranslationROffset=0  TranslationROffsetUnits=m  TranslationThetaOffset=0  TranslationThetaOffsetUnits=deg  TranslationZOffset=0  TranslationZOffsetUnits=m
  RT ArmaSfGCS SLO : sm_lib/Frames and Transforms/Rigid Transform  RotationMethod=RotationSequence  FollAlignAxisA=+X  BaseAlignAxisA=+Y  FollAlignAxisB=+Y  BaseAlignAxisB=+Z  RotationStandardAxis=+Z  RotationAngle=0  RotationAngleUnits=deg  RotationArbitraryAxis=[0 0 1]  RotationSequenceAxes=FollowerAxes  RotationSequence=ZYX  RotationSequenceAngles=ArmaSfCS_RA.SLO  RotationSequenceAnglesUnits=rad  RotationMatrix=[1 0 0;0 1 0;0 0 1]  Quaternion=[1 0 0 0]  TranslationMethod=StandardAxis  TranslationCartesianOffset=[0 0 0]  TranslationCartesianOffsetUnits=m  TranslationStandardAxis=+Y  TranslationStandardOffset=ArmaSfCS_Y_Off  TranslationStandardOffsetUnits=mm  TranslationROffset=0  TranslationROffsetUnits=m  TranslationThetaOffset=0  TranslationThetaOffsetUnits=deg  TranslationZOffset=0  TranslationZOffsetUnits=m
  RT ArmaSfGCS SLU : sm_lib/Frames and Transforms/Rigid Transform  RotationMethod=RotationSequence  FollAlignAxisA=+X  BaseAlignAxisA=+Y  FollAlignAxisB=+Y  BaseAlignAxisB=+Z  RotationStandardAxis=+Z  RotationAngle=0  RotationAngleUnits=deg  RotationArbitraryAxis=[0 0 1]  RotationSequenceAxes=FollowerAxes  RotationSequence=ZYX  RotationSequenceAngles=ArmaSfCS_RA.SLU  RotationSequenceAnglesUnits=rad  RotationMatrix=[1 0 0;0 1 0;0 0 1]  Quaternion=[1 0 0 0]  TranslationMethod=StandardAxis  TranslationCartesianOffset=[0 0 0]  TranslationCartesianOffsetUnits=m  TranslationStandardAxis=+Y  TranslationStandardOffset=ArmaSfCS_Y_Off  TranslationStandardOffsetUnits=mm  TranslationROffset=0  TranslationROffsetUnits=m  TranslationThetaOffset=0  TranslationThetaOffsetUnits=deg  TranslationZOffset=0  TranslationZOffsetUnits=m
  RT ArmaSfGCS SRO : sm_lib/Frames and Transforms/Rigid Transform  RotationMethod=RotationSequence  FollAlignAxisA=+X  BaseAlignAxisA=+Y  FollAlignAxisB=+Y  BaseAlignAxisB=+Z  RotationStandardAxis=+Z  RotationAngle=0  RotationAngleUnits=deg  RotationArbitraryAxis=[0 0 1]  RotationSequenceAxes=FollowerAxes  RotationSequence=ZYX  RotationSequenceAngles=ArmaSfCS_RA.SRO  RotationSequenceAnglesUnits=rad  RotationMatrix=[1 0 0;0 1 0;0 0 1]  Quaternion=[1 0 0 0]  TranslationMethod=StandardAxis  TranslationCartesianOffset=[0 0 0]  TranslationCartesianOffsetUnits=m  TranslationStandardAxis=+Y  TranslationStandardOffset=ArmaSfCS_Y_Off  TranslationStandardOffsetUnits=mm  TranslationROffset=0  TranslationROffsetUnits=m  TranslationThetaOffset=0  TranslationThetaOffsetUnits=deg  TranslationZOffset=0  TranslationZOffsetUnits=m
  RT ArmaSfGCS SRU : sm_lib/Frames and Transforms/Rigid Transform  RotationMethod=RotationSequence  FollAlignAxisA=+X  BaseAlignAxisA=+Y  FollAlignAxisB=+Y  BaseAlignAxisB=+Z  RotationStandardAxis=+Z  RotationAngle=0  RotationAngleUnits=deg  RotationArbitraryAxis=[0 0 1]  RotationSequenceAxes=FollowerAxes  RotationSequence=ZYX  RotationSequenceAngles=ArmaSfCS_RA.SRU  RotationSequenceAnglesUnits=rad  RotationMatrix=[1 0 0;0 1 0;0 0 1]  Quaternion=[1 0 0 0]  TranslationMethod=StandardAxis  TranslationCartesianOffset=[0 0 0]  TranslationCartesianOffsetUnits=m  TranslationStandardAxis=+Y  TranslationStandardOffset=ArmaSfCS_Y_Off  TranslationStandardOffsetUnits=mm  TranslationROffset=0  TranslationROffsetUnits=m  TranslationThetaOffset=0  TranslationThetaOffsetUnits=deg  TranslationZOffset=0  TranslationZOffsetUnits=m
  Arma_Poleface ELO : PMIOPort  Side=Right
  Arma_Poleface ERO : PMIOPort  Port=2  Side=Right
  Arma_Poleface ELU : PMIOPort  Port=3  Side=Right
  Arma_Poleface ERU : PMIOPort  Port=4  Side=Right
  Arma_Poleface SLO : PMIOPort  Port=5  Side=Left
  Arma_Poleface SRO : PMIOPort  Port=6  Side=Left
  Arma_Poleface SLU : PMIOPort  Port=7  Side=Left
  Arma_Poleface SRU : PMIOPort  Port=8  Side=Left
  B : PMIOPort  Port=9  Side=Left
  connections:
  GCRLW2MDRCS/LConn1 -- MDRCS2WD/RConn1
  MDRCS2WD/LConn1 -- B/RConn1
  Arma_Poleface ELO/RConn1 -- RT ArmaSfGCS ELO/RConn1
  Armature ERO/RConn1 -- RT ArmaSfGCS ERO/LConn1 -- RT ArmaGCS ERO/RConn1
  Armature SLO/RConn1 -- RT ArmaSfGCS SLO/LConn1 -- RT ArmaGCS SLO/RConn1
  RT ArmaGCS SRO/RConn1 -- RT ArmaSfGCS SRO/LConn1 -- Armature SRO/RConn1
  RT ArmaSfGCS ELU/LConn1 -- Armature ELU/RConn1 -- RT ArmaGCS ELU/RConn1
  Armature ERU/RConn1 -- RT ArmaSfGCS ERU/LConn1 -- RT ArmaGCS ERU/RConn1
  Armature SLU/RConn1 -- RT ArmaSfGCS SLU/LConn1 -- RT ArmaGCS SLU/RConn1
  Armature SRU/RConn1 -- RT ArmaSfGCS SRU/LConn1 -- RT ArmaGCS SRU/RConn1
  Arma_Poleface ERO/RConn1 -- RT ArmaSfGCS ERO/RConn1
  Arma_Poleface ELU/RConn1 -- RT ArmaSfGCS ELU/RConn1
  Arma_Poleface ERU/RConn1 -- RT ArmaSfGCS ERU/RConn1
  Arma_Poleface SLO/RConn1 -- RT ArmaSfGCS SLO/RConn1
  Arma_Poleface SRO/RConn1 -- RT ArmaSfGCS SRO/RConn1
  Arma_Poleface SLU/RConn1 -- RT ArmaSfGCS SLU/RConn1
  Arma_Poleface SRU/RConn1 -- RT ArmaSfGCS SRU/RConn1
  Machine Frame/RConn1 -- RT ArmaGCS SLU/LConn1 -- RT ArmaGCS SLO/LConn1 -- GCRLW2MDRCS/RConn1 -- RT ArmaGCS ELU/LConn1 -- RT ArmaGCS ELO/LConn1 -- RT ArmaGCS ERU/LConn1 -- RT ArmaGCS ERO/LConn1 -- RT ArmaGCS SRU/LConn1 -- RT ArmaGCS SRO/LConn1
  Armature ELO/RConn1 -- RT ArmaSfGCS ELO/LConn1 -- RT ArmaGCS ELO/RConn1
